simulink model "Assignment2SIMv3"  (R2023b)
settings: Solver=VariableStepAuto  StartTime=0.0  StopTime=6  RelTol=1e-3
libraries: simulink x2
settings Model: Creator=Mathias  LastModifiedBy=Mathias

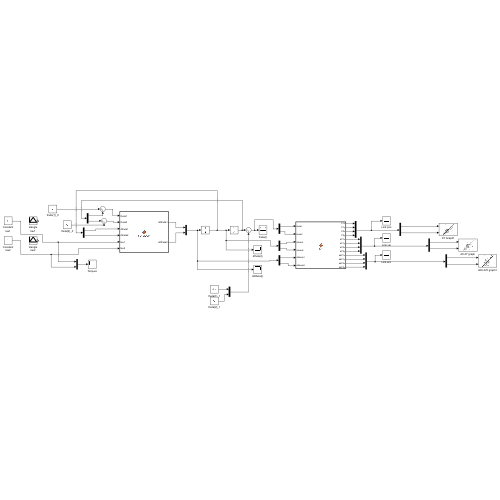
[thumbnail: Simulink's stored preview of the top-level diagram]
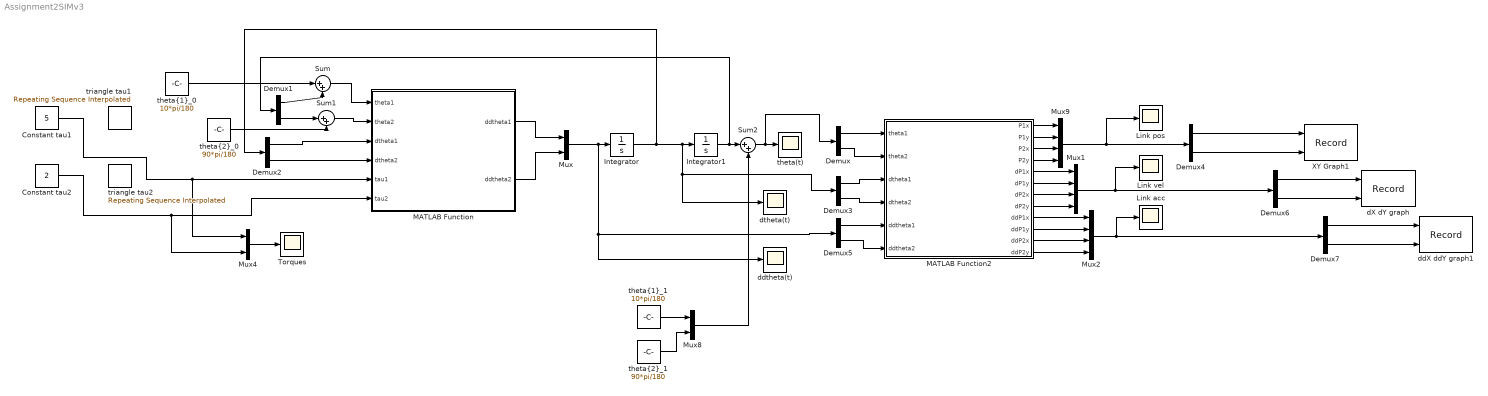
== system Assignment2SIMv3 ==
  Constant tau1 : Constant  Value=5
  Constant tau2 : Constant  Value=2
  Demux{,1..7} (8 alike) : Demux  Outputs=2
  Integrator : Integrator
  Integrator1 : Integrator
  Link acc : Scope
  Link pos : Scope
  Link vel : Scope
  MATLAB Function : MATLAB Function  TreatAsAtomicUnit=on
  MATLAB Function2 : MATLAB Function  TreatAsAtomicUnit=on
  Mux : Mux  Inputs=2
  Mux1 : Mux
  Mux2 : Mux
  Mux4 : Mux  Inputs=2
  Mux8 : Mux  Inputs=2
  Mux9 : Mux
  Sum : Sum  Inputs=|++
  Sum1 : Sum  Inputs=|++
  Sum2 : Sum  Inputs=|++
  Torques : Scope
  XY Graph1 : Record  FileSettingsInternal="{\"entries\":[{\"content\":{\"excelSettings\":{\"content\":{},\"type\":\"Streamout.ExcelSettings\"}},\"type\":\"Streamout.FileSettingStorage\",\"uuid\":\"\"}],\"packageUris\":[\"http:\\/\\/schema.mathworks.com\\/mf0\\/streamout_blocks\\/R2020a\"],\"version\":\"1.0\"}"  Layout=[1 1]  SignalsInternal="{\"entries\":[{\"content\":{\"signals\":[{\"content\":{\"blockPath\":[],\"dimensions\":[2],\"domain\":\"\",\"hasChildren\":true,\"lineColor\":\"#64d413\",\"port\":1,\"sid\":[\"\"],\"signalID\":1,\"signalName\":\"Demux4:1\"},\"type\":\"RecordBlkView.Signal\",\"uuid\":\"\"},{\"content\":{\"blockPath\":[],\"channel\":[1],\"dimensions\":[2],\"domain\":\"\",\"lineColor\":\"#7e2f8e\",\"parentID\":1,\"plots\":[ 1 ],\"port\":1,\"sid\":[\"\"],\"signalID\":2,\"signalName\":\"Demux4:1\"},\"type\":\"RecordBlkView.Signal\",\"uuid\":\"\"},{\"content\":{\"blockPath\":[],\"dimensions\":[2],\"domain\":\"\",\"hasChildren\":true,\"lineColor\":\"#fe330a\",\"port\":2,\"sid\":[\"\"],\"signalID\":3,\"signalName\":\"Demux4:2\"},\"type\":\"RecordBlkView.Signal\",\"uuid\":\"\"},{\"content\":{\"blockPath\":[],\"channel\":[1],\"dimensions\":[2],\"domain\":\"\",\"lineColor\":\"#4dbeee\",\"parentID\":3,\"plots\":[ 1 ],\"port\":2,\"sid\":[\"\"],\"signalID\":4,\"signalName\":\"Demux4:2\"},\"type\":\"RecordBlkView.Signal\",\"uuid\":\"\"},{\"content\":{\"blockPath\":[],\"channel\":[2],\"dimensions\":[2],\"domain\":\"\",\"lineColor\":\"#64d413\",\"parentID\":1,\"plots\":[ 1 ],\"port\":1,\"sid\":[\"\"],\"signalID\":5,\"signalName\":\"Demux4:1\"},\"type\":\"RecordBlkView.Signal\",\"uuid\":\"\"},{\"content\":{\"blockPath\":[],\"channel\":[2],\"dimensions\":[2],\"domain\":\"\",\"lineColor\":\"#ff13a6\",\"parentID\":3,\"plots\":[ 1 ],\"port\":2,\"sid\":[\"\"],\"signalID\":6,\"signalName\":\"Demux4:2\"},\"type\":\"RecordBlkView.Signal\",\"uuid\":\"\"}]},\"type\":\"RecordBlkView.InputSignals\",\"uuid\":\"\"}],\"packageUris\":[\"http:\\/\\/schema.mathworks.com\\/mf0\\/streamout_blocks\\/R2020a\"],\"version\":\"1.0\"}"  VisualizationBindings="{\"xyplotplugin\":{\"info\":[{\"series\":[{\"bindingParametersList\":[{\"parameter\":\"X-Axis\",\"signalID\":4,\"signalName\":\"Demux4:2(1)\"},{\"parameter\":\"Y-Axis\",\"signalID\":6,\"signalName\":\"Demux4:2(2)\"}],\"seriesID\":0},{\"bindingParametersList\":[{\"parameter\":\"X-Axis\",\"signalID\":2,\"signalName\":\"Demux4:1(1)\"},{\"parameter\":\"Y-Axis\",\"signalID\":5,\"signalName\":\"Demux4:1(2)\"}],\"seriesID\":1}],\"subplotID\":1}]}}"  CompatibilityTag=XY
  dX dY graph : Record  FileSettingsInternal="{\"entries\":[{\"content\":{\"excelSettings\":{\"content\":{},\"type\":\"Streamout.ExcelSettings\"}},\"type\":\"Streamout.FileSettingStorage\",\"uuid\":\"\"}],\"packageUris\":[\"http:\\/\\/schema.mathworks.com\\/mf0\\/streamout_blocks\\/R2020a\"],\"version\":\"1.0\"}"  Layout=[1 1]  SignalsInternal="{\"entries\":[{\"content\":{\"signals\":[{\"content\":{\"blockPath\":[],\"dimensions\":[2],\"domain\":\"\",\"hasChildren\":true,\"lineColor\":\"#0072bd\",\"port\":1,\"sid\":[\"\"],\"signalID\":1,\"signalName\":\"Demux6:1\"},\"type\":\"RecordBlkView.Signal\",\"uuid\":\"\"},{\"content\":{\"blockPath\":[],\"channel\":[1],\"dimensions\":[2],\"domain\":\"\",\"lineColor\":\"#7e2f8e\",\"parentID\":1,\"plots\":[ 1 ],\"port\":1,\"sid\":[\"\"],\"signalID\":2,\"signalName\":\"Demux6:1\"},\"type\":\"RecordBlkView.Signal\",\"uuid\":\"\"},{\"content\":{\"blockPath\":[],\"dimensions\":[2],\"domain\":\"\",\"hasChildren\":true,\"lineColor\":\"#edb120\",\"port\":2,\"sid\":[\"\"],\"signalID\":3,\"signalName\":\"Demux6:2\"},\"type\":\"RecordBlkView.Signal\",\"uuid\":\"\"},{\"content\":{\"blockPath\":[],\"channel\":[1],\"dimensions\":[2],\"domain\":\"\",\"lineColor\":\"#4dbeee\",\"parentID\":3,\"plots\":[ 1 ],\"port\":2,\"sid\":[\"\"],\"signalID\":4,\"signalName\":\"Demux6:2\"},\"type\":\"RecordBlkView.Signal\",\"uuid\":\"\"},{\"content\":{\"blockPath\":[],\"channel\":[2],\"dimensions\":[2],\"domain\":\"\",\"lineColor\":\"#64d413\",\"parentID\":1,\"plots\":[ 1 ],\"port\":1,\"sid\":[\"\"],\"signalID\":5,\"signalName\":\"Demux6:1\"},\"type\":\"RecordBlkView.Signal\",\"uuid\":\"\"},{\"content\":{\"blockPath\":[],\"channel\":[2],\"dimensions\":[2],\"domain\":\"\",\"lineColor\":\"#ff13a6\",\"parentID\":3,\"plots\":[ 1 ],\"port\":2,\"sid\":[\"\"],\"signalID\":6,\"signalName\":\"Demux6:2\"},\"type\":\"RecordBlkView.Signal\",\"uuid\":\"\"}]},\"type\":\"RecordBlkView.InputSignals\",\"uuid\":\"\"}],\"packageUris\":[\"http:\\/\\/schema.mathworks.com\\/mf0\\/streamout_blocks\\/R2020a\"],\"version\":\"1.0\"}"  VisualizationBindings="{\"xyplotplugin\":{\"info\":[{\"series\":[{\"bindingParametersList\":[{\"parameter\":\"X-Axis\",\"signalID\":2,\"signalName\":\"Demux6:1(1)\"},{\"parameter\":\"Y-Axis\",\"signalID\":5,\"signalName\":\"Demux6:1(2)\"}],\"seriesID\":0},{\"bindingParametersList\":[{\"parameter\":\"X-Axis\",\"signalID\":4,\"signalName\":\"Demux6:2(1)\"},{\"parameter\":\"Y-Axis\",\"signalID\":6,\"signalName\":\"Demux6:2(2)\"}],\"seriesID\":1}],\"subplotID\":1}]}}"  CompatibilityTag=XY
  ddX ddY graph1 : Record  FileSettingsInternal="{\"entries\":[{\"content\":{\"excelSettings\":{\"content\":{},\"type\":\"Streamout.ExcelSettings\"}},\"type\":\"Streamout.FileSettingStorage\",\"uuid\":\"\"}],\"packageUris\":[\"http:\\/\\/schema.mathworks.com\\/mf0\\/streamout_blocks\\/R2020a\"],\"version\":\"1.0\"}"  Layout=[1 1]  SignalsInternal="{\"entries\":[{\"content\":{\"signals\":[{\"content\":{\"blockPath\":[],\"dimensions\":[2],\"domain\":\"\",\"hasChildren\":true,\"lineColor\":\"#77ac30\",\"port\":1,\"sid\":[\"\"],\"signalID\":1,\"signalName\":\"Demux7:1\"},\"type\":\"RecordBlkView.Signal\",\"uuid\":\"\"},{\"content\":{\"blockPath\":[],\"channel\":[1],\"dimensions\":[2],\"domain\":\"\",\"lineColor\":\"#139fff\",\"parentID\":1,\"plots\":[ 1 ],\"port\":1,\"sid\":[\"\"],\"signalID\":2,\"signalName\":\"Demux7:1\"},\"type\":\"RecordBlkView.Signal\",\"uuid\":\"\"},{\"content\":{\"blockPath\":[],\"dimensions\":[2],\"domain\":\"\",\"hasChildren\":true,\"lineColor\":\"#a2142f\",\"port\":2,\"sid\":[\"\"],\"signalID\":3,\"signalName\":\"Demux7:2\"},\"type\":\"RecordBlkView.Signal\",\"uuid\":\"\"},{\"content\":{\"blockPath\":[],\"channel\":[1],\"dimensions\":[2],\"domain\":\"\",\"lineColor\":\"#b746ff\",\"parentID\":3,\"plots\":[ 1 ],\"port\":2,\"sid\":[\"\"],\"signalID\":4,\"signalName\":\"Demux7:2\"},\"type\":\"RecordBlkView.Signal\",\"uuid\":\"\"},{\"content\":{\"blockPath\":[],\"channel\":[2],\"dimensions\":[2],\"domain\":\"\",\"lineColor\":\"#0072bd\",\"parentID\":1,\"plots\":[ 1 ],\"port\":1,\"sid\":[\"\"],\"signalID\":5,\"signalName\":\"Demux7:1\"},\"type\":\"RecordBlkView.Signal\",\"uuid\":\"\"},{\"content\":{\"blockPath\":[],\"channel\":[2],\"dimensions\":[2],\"domain\":\"\",\"lineColor\":\"#d95319\",\"parentID\":3,\"plots\":[ 1 ],\"port\":2,\"sid\":[\"\"],\"signalID\":6,\"signalName\":\"Demux7:2\"},\"type\":\"RecordBlkView.Signal\",\"uuid\":\"\"}]},\"type\":\"RecordBlkView.InputSignals\",\"uuid\":\"\"}],\"packageUris\":[\"http:\\/\\/schema.mathworks.com\\/mf0\\/streamout_blocks\\/R2020a\"],\"version\":\"1.0\"}"  VisualizationBindings="{\"xyplotplugin\":{\"info\":[{\"series\":[{\"bindingParametersList\":[{\"parameter\":\"X-Axis\",\"signalID\":2,\"signalName\":\"Demux7:1(1)\"},{\"parameter\":\"Y-Axis\",\"signalID\":5,\"signalName\":\"Demux7:1(2)\"}],\"seriesID\":0},{\"bindingParametersList\":[{\"parameter\":\"X-Axis\",\"signalID\":4,\"signalName\":\"Demux7:2(1)\"},{\"parameter\":\"Y-Axis\",\"signalID\":6,\"signalName\":\"Demux7:2(2)\"}],\"seriesID\":1}],\"subplotID\":1}]}}"  CompatibilityTag=XY
  ddtheta(t) : Scope
  dtheta(t) : Scope
  theta(t) : Scope
  "theta{1}_0" : Constant  Value=10*pi/180
  "theta{1}_1" : Constant  Value=10*pi/180
  "theta{2}_0" : Constant  Value=90*pi/180
  "theta{2}_1" : Constant  Value=90*pi/180
  triangle tau1 : simulink/Sources/Repeating Sequence Interpolated  OutValues=[0 6 0].'  TimeValues=[0 3 6].'  LookUpMeth=Interpolation-Use End Values  tsamp=0.001  OutMin=[]  OutMax=[]  OutDataTypeStr=double  OutputDataTypeScalingMode=double  OutDataType=fixdt(0,8)  OutScaling=2^-10
  triangle tau2 : simulink/Sources/Repeating Sequence Interpolated  OutValues=[0 3.5 0].'  TimeValues=[0 3 6].'  LookUpMeth=Interpolation-Use End Values  tsamp=0.001  OutMin=[]  OutMax=[]  OutDataTypeStr=double  OutputDataTypeScalingMode=double  OutDataType=fixdt(0,8)  OutScaling=2^-10
  wires:
  Demux2/2 -> MATLAB Function/4(dtheta2)
  MATLAB Function/2(ddtheta2) -> Mux/2
  Demux2/1 -> MATLAB Function/3(dtheta1)
  Integrator/1 -> Demux2/1, Demux3/1, dtheta(t)/1, Integrator1/1
  MATLAB Function/1(ddtheta1) -> Mux/1
  Mux/1 -> Demux5/1, ddtheta(t)/1, Integrator/1
  Integrator1/1 -> Demux1/1, Sum2/1
  Mux4/1 -> Torques/1
  Demux/1 -> MATLAB Function2/1(theta1)
  Demux/2 -> MATLAB Function2/2(theta2)
  Demux3/1 -> MATLAB Function2/3(dtheta1)
  Demux3/2 -> MATLAB Function2/4(dtheta2)
  Demux5/1 -> MATLAB Function2/5(ddtheta1)
  Demux5/2 -> MATLAB Function2/6(ddtheta2)
  Demux1/1 -> Sum/2
  Sum/1 -> MATLAB Function/1(theta1)
  "theta{1}_0"/1 -> Sum/1
  Demux1/2 -> Sum1/1
  Sum1/1 -> MATLAB Function/2(theta2)
  "theta{2}_0"/1 -> Sum1/2
  Mux8/1 -> Sum2/2
  Sum2/1 -> Demux/1, theta(t)/1
  "theta{2}_1"/1 -> Mux8/2
  "theta{1}_1"/1 -> Mux8/1
  MATLAB Function2/1(P1x) -> Mux9/1
  MATLAB Function2/2(P1y) -> Mux9/2
  MATLAB Function2/3(P2x) -> Mux9/3
  MATLAB Function2/4(P2y) -> Mux9/4
  Demux4/2 -> XY Graph1/2
  Demux4/1 -> XY Graph1/1
  Mux9/1 -> Link pos/1, Demux4/1
  MATLAB Function2/5(dP1x) -> Mux1/1
  MATLAB Function2/6(dP1y) -> Mux1/2
  MATLAB Function2/7(dP2x) -> Mux1/3
  MATLAB Function2/8(dP2y) -> Mux1/4
  Demux6/2 -> dX dY graph/2
  Demux6/1 -> dX dY graph/1
  Mux1/1 -> Link vel/1, Demux6/1
  MATLAB Function2/9(ddP1x) -> Mux2/1
  MATLAB Function2/10(ddP1y) -> Mux2/2
  MATLAB Function2/11(ddP2x) -> Mux2/3
  MATLAB Function2/12(ddP2y) -> Mux2/4
  Demux7/1 -> ddX ddY graph1/1
  Demux7/2 -> ddX ddY graph1/2
  Mux2/1 -> Link acc/1, Demux7/1
  Constant tau1/1 -> Mux4/1, MATLAB Function/5(tau1)
  Constant tau2/1 -> Mux4/2, MATLAB Function/6(tau2)

== matlab function Assignment2SIMv3/MATLAB Function ==
  data: theta1 input; theta2 input; dtheta1 input; dtheta2 input; tau1 input; ddtheta1 output; tau2 input; ddtheta2 output
function [ddtheta1, ddtheta2] = FD_2DOF(theta1, theta2, dtheta1, dtheta2, tau1, tau2) % , ddtheta2]
% ============================== %
% Initialize provided parameters %
% ============================== %
l = [ 1.0, 0.5 ]; % Link length
m = [ 19.5, 9.75 ]; % Link mass
c = [ l(1)/2, l(2)/2 ]; % mass center
I = [ 1/3 * m(1) * l(1)^2, 1/3 * m(2) * l(2)^2 ]; % moment of inertia
g = 9.801; % Gravity constant

%{
% Coefficients of dynamic equation
H11 = m(1)*c(1)^2 + I(1) + m(2)*(l(1)^2 + c(2)^2 + 2*l(1)*c(2)*cos(theta2)) + I(2);
H22 = m(2)*c(2)^2 + I(2); 
H12 = m(2)*(c(2)^2 + l(1)*c(2)*cos(theta2)) + I(2); 
h = m(2)*l(1)*c(2)*sin(theta2); 
G1 = m(1)*c(1)*g*cos(theta1) ...
        + m(2)*g*(c(2)*cos(theta1 + theta2) + l(1)*cos(theta1)); 
G2 = m(2)*g*c(2)*cos(theta1 + theta2);
%}
H12 = m(2)*l(1)*c(2)*cos(theta2) + I(2); 
H11 = I(1) + m(2)*(l(1)^2 + l(1)*c(2)*cos(theta2)) + H12;
H22 = I(2); 

h = m(2)*c(2)*sin(theta2);
G1 = m(1)*g*c(1)*cos(theta1) + m(2)*g*( c(2)*cos(theta1 + theta2) + l(1) * cos(theta1 ) ); 
G2 = m(2)*g*c(2)*cos(theta1 + theta2);

% Matrix depicting the non-zero coefficients of dynamic equation
H = [H11 H12;
     H12 H22];
V = [h*(dtheta2)^2 - 2*h*dtheta1*dtheta2, h*(theta1)^2];
G = [G1; G2];

ddtheta = H \ ([tau1; tau2] - (V + G));
[ddtheta1, ddtheta2] = deal(ddtheta(1), ddtheta(2));

== matlab function Assignment2SIMv3/MATLAB Function2 ==
  data: theta1 input; P1x output; theta2 input; P1y output; P2x output; P2y output; dtheta1 input; dtheta2 input; dP1x output; dP1y output; dP2x output; dP2y output; ddtheta1 input; ddtheta2 input; ddP1x output; ddP1y output; ddP2x output; ddP2y output
function [P1x, P1y, P2x, P2y, dP1x, dP1y, dP2x, dP2y, ddP1x, ddP1y, ddP2x, ddP2y] = fcn(theta1, theta2, dtheta1, dtheta2, ddtheta1, ddtheta2)

% ============================== %
% Initialize provided parameters %
% ============================== %
l = [ 1.0, 0.5 ]; % Link length

s_1 = [ % Link 0->1 position vector
    l(1) * cos(theta1);                    % s_1{1}(t)
    l(1) * sin(theta1);                    % s_1{2}(t)
    0
];
s_2 = [ % Link 1->2 position vector
    l(2) * cos(theta1 + theta2);   % s_2{1}(t)
    l(2) * sin(theta1 + theta2);   % s_2{2}(t)
    0
];

[ P1x, P1y ]  = deal(s_1(1), s_1(2));
[ P2x, P2y ] = deal(P1x + s_2(1), P1y + s_2(2));

% ========================================================= %
% Get link position, velocity, and acceleration             %
% using recursive method.                                   %
% ========================================================= %
% The alternative is to get Jacobian J and its time         %
% derivative dJ, yet this requires more processes compared  %
% to using recursive method.                                %
% ========================================================= %
[ omega_1, domega_1 ] = deal([ 0; 0; dtheta1 ], [ 0; 0; ddtheta1 ]);
[ omega_2, domega_2 ] = deal(omega_1 + [ 0; 0; dtheta2 ], domega_1 + [ 0; 0; ddtheta2 ]);

% Get link 1 velocity and acceleration function
v_1 = cross(omega_1, s_1);
a_1 = cross(domega_1, s_1) + cross(omega_1, cross(omega_1, s_1));

% Get link 2 velocity and acceleration
v_2 = v_1 + cross(omega_2, s_2);
a_2 = a_1 + cross(domega_2, s_2) + cross(omega_2, cross(omega_2, s_2));

[ dP1x, dP1y ] = deal(v_1(1), v_1(2)); % dx/dt
[ dP2x, dP2y ] = deal(v_2(1), v_2(2)); % dx/dt

[ ddP1x, ddP1y ] = deal(a_1(1), a_1(2)); % d^2x/dt^2
[ ddP2x, ddP2y ] = deal(a_2(1), a_2(2)); % d^2x/dt^2
